simulink model "dynamics"  (R2025b)
settings: Solver=VariableStepAuto  StartTime=0.0  StopTime=10.0  RelTol=1e-3
settings Model: Creator=samue  LastModifiedBy=samue

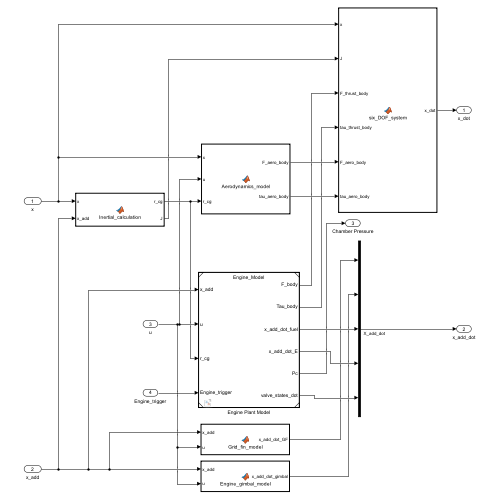
[thumbnail: Simulink's stored preview of the top-level diagram]
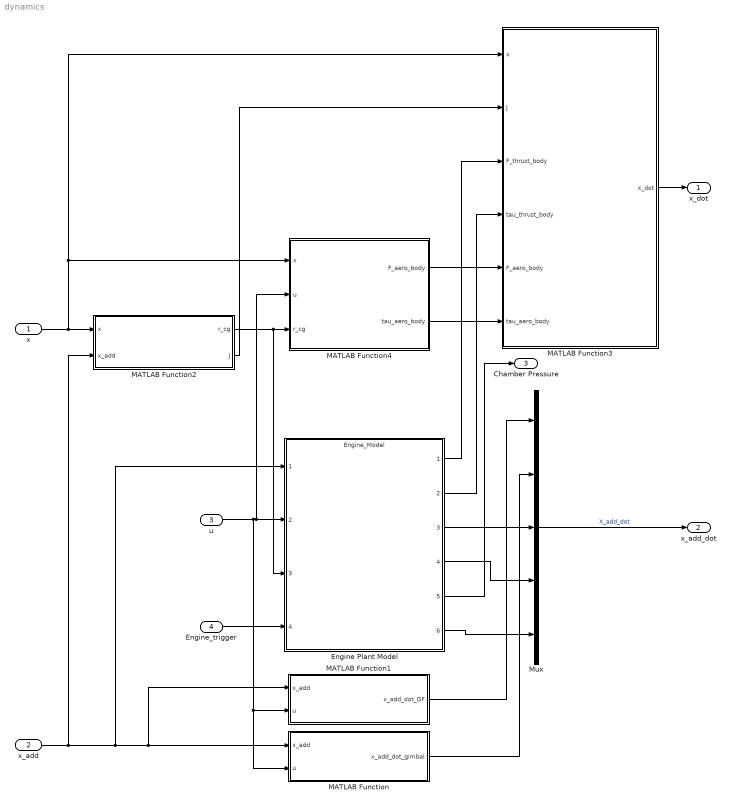
== system dynamics ==
  x : Inport
  x_add : Inport  Port=2
  u : Inport  Port=3
  Engine_trigger : Inport  Port=4
  Engine Plant Model : ModelReference  ModelNameDialog=Engine_Model.slx  SimulationMode=Normal  ModelReferenceVersion=1.43
  MATLAB Function : MATLAB Function  TreatAsAtomicUnit=on
  MATLAB Function1 : MATLAB Function  TreatAsAtomicUnit=on
  MATLAB Function2 : MATLAB Function  TreatAsAtomicUnit=on
  MATLAB Function3 : MATLAB Function  TreatAsAtomicUnit=on
  MATLAB Function4 : MATLAB Function  TreatAsAtomicUnit=on
  Mux : Mux  Inputs=5
  x_dot : Outport
  x_add_dot : Outport  Port=2
  Chamber Pressure : Outport  Port=3
  wires:
  x/1 -> MATLAB Function4/1(x), MATLAB Function3/1(x), MATLAB Function2/1(x)
  MATLAB Function3/1(x_dot) -> x_dot/1
  x_add/1 -> MATLAB Function/1(x_add), MATLAB Function1/1(x_add), Engine Plant Model/1, MATLAB Function2/2(x_add)
  u/1 -> MATLAB Function/2(u), MATLAB Function1/2(u), MATLAB Function4/2(u), Engine Plant Model/2
  Engine_trigger/1 -> Engine Plant Model/4
  MATLAB Function2/2(J) -> MATLAB Function3/2(J)
  MATLAB Function2/1(r_cg) -> MATLAB Function4/3(r_cg), Engine Plant Model/3
  MATLAB Function4/1(F_aero_body) -> MATLAB Function3/5(F_aero_body)
  MATLAB Function4/2(tau_aero_body) -> MATLAB Function3/6(tau_aero_body)
  Engine Plant Model/1 -> MATLAB Function3/3(F_thrust_body)
  Engine Plant Model/2 -> MATLAB Function3/4(tau_thrust_body)
  Mux/1 -> x_add_dot/1  "X_add_dot"
  Engine Plant Model/3 -> Mux/3
  Engine Plant Model/4 -> Mux/4
  Engine Plant Model/5 -> Chamber Pressure/1
  Engine Plant Model/6 -> Mux/5
  MATLAB Function1/1(x_add_dot_GF) -> Mux/1
  MATLAB Function/1(x_add_dot_gimbal) -> Mux/2

== matlab function dynamics/MATLAB Function1 ==
  data: x_add input; u input; x_add_dot_GF output; config parameter
function x_add_dot_GF = Grid_fin_model(x_add, u, config)
% Grid fin actuator model to get state derivative
% x_add_GF = [theta_m, theta_m_dot, theta_L, theta_L_dot]
    % Initialise vector
    x_add_dot_GF = zeros(12, 1);

    % Loop through each grid fin and calculate state
    for i = 1:3
        actuator_state = x_add((2 + i) : (2 + 4 * i));
        x_add_dot_GF_i = GF_actuator_dynamic_fn(actuator_state, ...
            u(i), config);
        x_add_dot_GF((2 + 4 * (i - 1)) : (2 + 4 * i)) = x_add_dot_GF_i;
    end
end

== matlab function dynamics/MATLAB Function ==
  data: x_add input; u input; x_add_dot_gimbal output; config parameter
function x_add_dot_gimbal = Engine_gimbal_model(x_add, u, config)
% Calculate engine gimbal rate
    % gimbal_state = [alpha_y, alpha_y_dot, alpha_z, alpha_z_dot]
    gimbal_state = x_add(15:18);
    u_gimbal = u(4:5);
    [x_add_dot_gimbal] = Engine_gimbal_dynamics_fn(gimbal_state, ...
        u_gimbal, config);
end

== matlab function dynamics/MATLAB Function2 ==
  data: x input; r_cg output; x_add input; config parameter; J output
function [r_cg, J] = Inertial_calculation(x, x_add, config)
% Calculates 
    % Mass components
    m = x(14);
    m_fuel = x_add(1);
    m_ox = x_add(2);

    % Inertial_calculation
    [r_cg, J] = Get_inertia_and_mass(m, ...
        m_fuel, m_ox, config);
end

== matlab function dynamics/MATLAB Function3 ==
  data: x input; x_dot output; J input; F_thrust_body input; tau_thrust_body input; F_aero_body input; tau_aero_body input; config parameter
function x_dot  = six_DOF_system(x, ...
        J, F_thrust_body, tau_thrust_body, F_aero_body, ...
        tau_aero_body, config)
% Calculates state derivative with forces and torques
    x_dot = Get_state_derivative(x, ...
        J, F_thrust_body, tau_thrust_body, F_aero_body, ...
        tau_aero_body, config);
end

== matlab function dynamics/MATLAB Function4 ==
  data: x input; F_aero_body output; u input; r_cg input; config parameter; tau_aero_body output
function [F_aero_body, tau_aero_body] = Aerodynamics_model(x, u, r_cg, config)
% calculates aerodynamic forces and torques acting on the rocket in body axes
    % Take components out of inputs
    x_cg = r_cg(1);
    u_fins = u(1:3);

    % Calculate aerodynamic forces
    [F_aero_body, tau_aero_body] = Aerodynamic_forces(x, ...
        u_fins, x_cg, config);
end
